simulink model "untitled"  (R2024a)
settings: Solver=FixedStepAuto  StartTime=0.0  StopTime=900  FixedStep=0.001  RelTol=1e-3
model workspace (MAT data in the model file):
  time_delay1 = 0
settings Model: Creator=85063  LastModifiedBy=85063
settings DataIOCC: ExternalInput=sig1

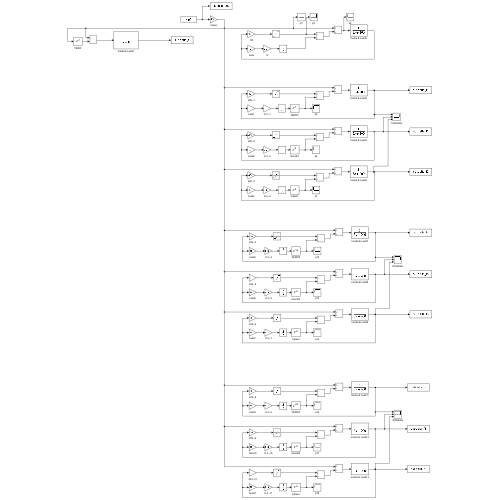
[thumbnail: Simulink's stored preview of the top-level diagram]
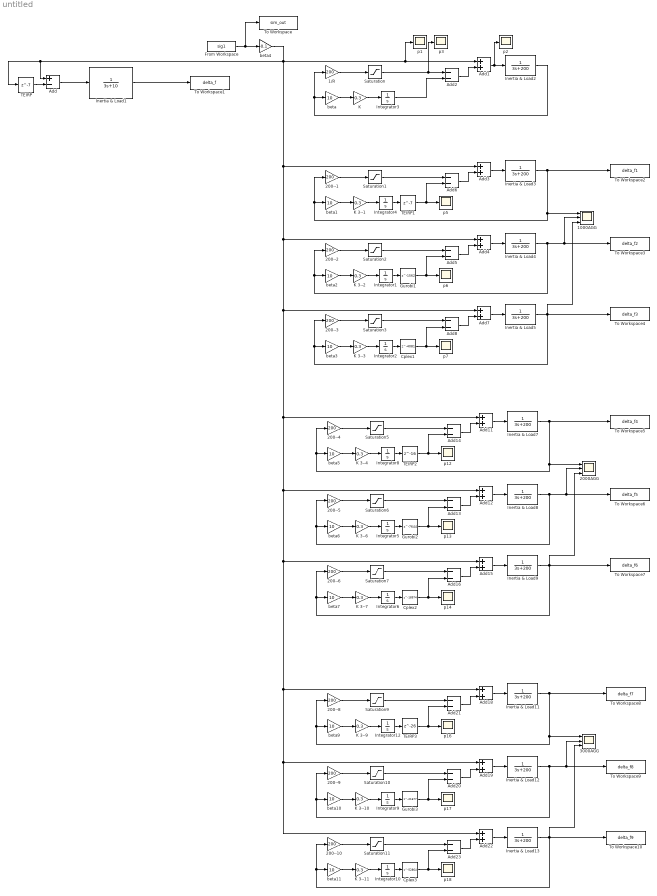
== system untitled ==
  1/R : Gain  Gain=200
  1000AGG : Scope  NumInputPorts=3
  200--{1..6,8..10} (9 alike) : Gain  Gain=200
  2000AGG : Scope  NumInputPorts=3
  3000AGG : Scope  NumInputPorts=3
  Add : Sum  Inputs=+-
  Add{1,3..4,7,11..12,15,18..19,22} (10 alike) : Sum
  Add{2,5..6,8,13..14,16,20..21,23} (10 alike) : Sum  Inputs=--
  Cplex1 : Delay  DelayLength=4081  InitialCondition=0
  Cplex2 : Delay  DelayLength=18974  InitialCondition=0
  Cplex3 : Delay  DelayLength=52864  InitialCondition=0
  From Workspace : FromWorkspace  VariableName=sig1  OutDataTypeStr=double  OutputAfterFinalValue=Holding final value
  Gurobi1 : Delay  DelayLength=1562  InitialCondition=0
  Gurobi2 : Delay  DelayLength=7644  InitialCondition=0
  Gurobi3 : Delay  DelayLength=21677  InitialCondition=0
  Inertia & Load1 : TransferFcn  Denominator=[3 10]
  Inertia & Load{2..5,7..9,11..13} (10 alike) : TransferFcn  Denominator=[3 200]
  Integrator{1..6,8..10,12} (10 alike) : Integrator
  K : Gain  Gain=0.3
  K 3--{1..4,6..7,9..11} (9 alike) : Gain  Gain=0.3
  Saturation{,1..3,5..7,9..11} (10 alike) : Saturate  UpperLimit=2  LowerLimit=-2
  TEIRP : Delay  DelayLength=7  InitialCondition=0
  TEIRP1 : Delay  DelayLength=7  InitialCondition=0
  TEIRP2 : Delay  DelayLength=16  InitialCondition=0
  TEIRP3 : Delay  DelayLength=26  InitialCondition=0
  To Workspace : ToWorkspace  VariableName=sim_out  SampleTime=-1
  To Workspace1 : ToWorkspace  VariableName=delta_f  SampleTime=-1
  To Workspace10 : ToWorkspace  VariableName=delta_f9  SampleTime=-1
  To Workspace2 : ToWorkspace  VariableName=delta_f1  SampleTime=-1
  To Workspace3 : ToWorkspace  VariableName=delta_f2  SampleTime=-1
  To Workspace4 : ToWorkspace  VariableName=delta_f3  SampleTime=-1
  To Workspace5 : ToWorkspace  VariableName=delta_f4  SampleTime=-1
  To Workspace6 : ToWorkspace  VariableName=delta_f5  SampleTime=-1
  To Workspace7 : ToWorkspace  VariableName=delta_f6  SampleTime=-1
  To Workspace8 : ToWorkspace  VariableName=delta_f7  SampleTime=-1
  To Workspace9 : ToWorkspace  VariableName=delta_f8  SampleTime=-1
  beta{,1..3,5..7,9..11} (10 alike) : Gain  Gain=10
  beta4 : Gain  Gain=-0.1
  p{1..3,5..7,12..14,16..18} (12 alike) : Scope
  wires:
  Add/1 -> Inertia & Load1/1
  Inertia & Load1/1 -> To Workspace1/1
  TEIRP/1 -> Add/2
  Add1/1 -> p2/1, Inertia & Load2/1
  Add2/1 -> Add1/2
  1/R/1 -> Saturation/1
  beta/1 -> K/1
  K/1 -> Integrator3/1
  Saturation/1 -> p3/1, Add2/1
  Integrator3/1 -> Add2/2
  Inertia & Load2/1 -> 1/R/1, beta/1
  beta1/1 -> K 3--1/1
  200--1/1 -> Saturation1/1
  Saturation1/1 -> Add6/1
  Add6/1 -> Add3/2
  Integrator4/1 -> TEIRP1/1
  K 3--1/1 -> Integrator4/1
  Inertia & Load3/1 -> To Workspace2/1, 200--1/1, beta1/1, 1000AGG/1
  Add3/1 -> Inertia & Load3/1
  TEIRP1/1 -> p5/1, Add6/2
  Gurobi1/1 -> p6/1, Add5/2
  Add4/1 -> Inertia & Load4/1
  Inertia & Load4/1 -> 1000AGG/2, To Workspace3/1, 200--2/1, beta2/1
  Saturation2/1 -> Add5/1
  Integrator1/1 -> Gurobi1/1
  K 3--2/1 -> Integrator1/1
  200--2/1 -> Saturation2/1
  Add5/1 -> Add4/2
  beta2/1 -> K 3--2/1
  Saturation3/1 -> Add8/1
  200--3/1 -> Saturation3/1
  beta3/1 -> K 3--3/1
  Add8/1 -> Add7/2
  K 3--3/1 -> Integrator2/1
  Add7/1 -> Inertia & Load5/1
  Cplex1/1 -> p7/1, Add8/2
  Integrator2/1 -> Cplex1/1
  Inertia & Load5/1 -> To Workspace4/1, 200--3/1, beta3/1, 1000AGG/3
  TEIRP2/1 -> p12/1, Add14/2
  Add11/1 -> Inertia & Load7/1
  Saturation5/1 -> Add14/1
  Integrator8/1 -> TEIRP2/1
  beta6/1 -> K 3--6/1
  K 3--6/1 -> Integrator5/1
  Add14/1 -> Add11/2
  Add12/1 -> Inertia & Load8/1
  200--4/1 -> Saturation5/1
  Add13/1 -> Add12/2
  Add15/1 -> Inertia & Load9/1
  Saturation7/1 -> Add16/1
  beta7/1 -> K 3--7/1
  200--5/1 -> Saturation6/1
  200--6/1 -> Saturation7/1
  beta5/1 -> K 3--4/1
  Gurobi2/1 -> p13/1, Add13/2
  Add16/1 -> Add15/2
  Integrator5/1 -> Gurobi2/1
  K 3--7/1 -> Integrator6/1
  Cplex2/1 -> p14/1, Add16/2
  Integrator6/1 -> Cplex2/1
  Saturation6/1 -> Add13/1
  K 3--4/1 -> Integrator8/1
  K 3--9/1 -> Integrator12/1
  Add23/1 -> Add22/2
  Integrator9/1 -> Gurobi3/1
  Cplex3/1 -> p18/1, Add23/2
  Inertia & Load12/1 -> To Workspace9/1, 3000AGG/2, 200--9/1, beta10/1
  beta11/1 -> K 3--11/1
  Add22/1 -> Inertia & Load13/1
  Add20/1 -> Add19/2
  beta9/1 -> K 3--9/1
  Saturation10/1 -> Add20/1
  200--8/1 -> Saturation9/1
  200--10/1 -> Saturation11/1
  Add19/1 -> Inertia & Load12/1
  Gurobi3/1 -> p17/1, Add20/2
  200--9/1 -> Saturation10/1
  Add21/1 -> Add18/2
  Inertia & Load13/1 -> To Workspace10/1, 200--10/1, beta11/1, 3000AGG/3
  beta10/1 -> K 3--10/1
  Integrator10/1 -> Cplex3/1
  K 3--10/1 -> Integrator9/1
  Saturation9/1 -> Add21/1
  Integrator12/1 -> TEIRP3/1
  Saturation11/1 -> Add23/1
  K 3--11/1 -> Integrator10/1
  Add18/1 -> Inertia & Load11/1
  Inertia & Load11/1 -> 200--8/1, beta9/1, 3000AGG/1, To Workspace8/1
  TEIRP3/1 -> p16/1, Add21/2
  Inertia & Load9/1 -> To Workspace7/1, 200--6/1, beta7/1, 2000AGG/3
  Inertia & Load7/1 -> To Workspace5/1, 200--4/1, beta5/1, 2000AGG/1
  Inertia & Load8/1 -> 2000AGG/2, To Workspace6/1, 200--5/1, beta6/1
  beta4/1 -> Add/1, TEIRP/1, Add11/1, Add12/1, Add15/1, Add18/1, Add19/1, Add22/1, Add7/1, Add4/1, Add3/1, p1/1, Add1/1
  From Workspace/1 -> To Workspace/1, beta4/1
